simulink model "sml_trajectory"  (R2016a)
settings: Solver=VariableStepAuto  StartTime=0.0  StopTime=10.0  RelTol=1e-3
libraries: simulink x2
settings Model: Creator=Duy Nam  LastModifiedBy=Duy Nam

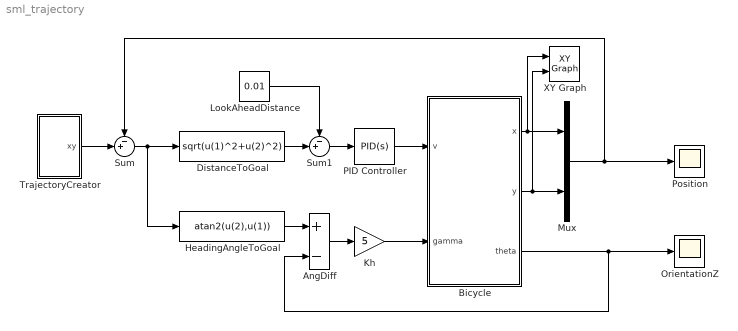
== system sml_trajectory ==
  AngDiff : Sum  Inputs=+-
  Bicycle : Subsystem
  DistanceToGoal : Fcn  Expr=sqrt(u(1)^2+u(2)^2)
  HeadingAngleToGoal : Fcn  Expr=atan2(u(2),u(1))
  Kh : Gain  Gain=5
  LookAheadDistance : Constant  Value=0.01
  Mux : Mux  Inputs=2
  OrientationZ : Scope
  PID Controller : simulink/Continuous/PID Controller  Controller=PID  TimeDomain=Continuous-time  SampleTime=-1  IntegratorMethod=Forward Euler  FilterMethod=Forward Euler  Form=Parallel  UseFilter=on  ControllerParametersSource=internal  P=4  I=0.5  D=0  N=100  InitialConditionSource=internal  InitialConditionForIntegrator=0  InitialConditionForFilter=0  ExternalReset=none  LimitOutput=off  UpperSaturationLimit=inf  LowerSaturationLimit=-inf  LinearizeAsGain=on  AntiWindupMode=none  Kb=1  TrackingMode=off  Kt=1  PParamMin=[]  PParamMax=[]  IParamMin=[]  IParamMax=[]  DParamMin=[]  DParamMax=[]  NParamMin=[]  NParamMax=[]  KbParamMin=[]  KbParamMax=[]  KtParamMin=[]  KtParamMax=[]  POutMin=[]  POutMax=[]  IOutMin=[]  IOutMax=[]  DOutMin=[]  DOutMax=[]  NOutMin=[]  NOutMax=[]  KbOutMin=[]  KbOutMax=[]  KtOutMin=[]  KtOutMax=[]  IntegratorOutMin=[]  IntegratorOutMax=[]  FilterOutMin=[]  FilterOutMax=[]  SumOutMin=[]  SumOutMax=[]  SumI1OutMin=[]  SumI1OutMax=[]  SumI2OutMin=[]  SumI2OutMax=[]  SumI3OutMin=[]  SumI3OutMax=[]  SumDOutMin=[]  SumDOutMax=[]  SaturationOutMin=[]  SaturationOutMax=[]  IntegratorContinuousStateAttributes=''  IntegratorStateMustResolveToSignalObject=off  IntegratorRTWStateStorageClass=Auto  FilterContinuousStateAttributes=''  FilterStateMustResolveToSignalObject=off  FilterRTWStateStorageClass=Auto  DifferentiatorICPrevScaledInput=0  DifferentiatorOutMin=[]  DifferentiatorOutMax=[]
  Position : Scope
  Sum : Sum  Inputs=-+|
  Sum1 : Sum  Inputs=-+|
  TrajectoryCreator : Subsystem
  XY Graph : simulink/Sinks/XY Graph  xmin=-5  xmax=5  ymin=-5  ymax=5  st=-1
  wires:
  Bicycle/1(x) -> XY Graph/1, Mux/1
  Bicycle/2(y) -> XY Graph/2, Mux/2
  Bicycle/3(theta) -> AngDiff/2, OrientationZ/1
  Mux/1 -> Sum/1, Position/1
  Sum/1 -> HeadingAngleToGoal/1, DistanceToGoal/1
  DistanceToGoal/1 -> Sum1/2
  LookAheadDistance/1 -> Sum1/1
  HeadingAngleToGoal/1 -> AngDiff/1
  Sum1/1 -> PID Controller/1
  AngDiff/1 -> Kh/1
  Kh/1 -> Bicycle/2(gamma)
  PID Controller/1 -> Bicycle/1(v)
  TrajectoryCreator/1(xy) -> Sum/2

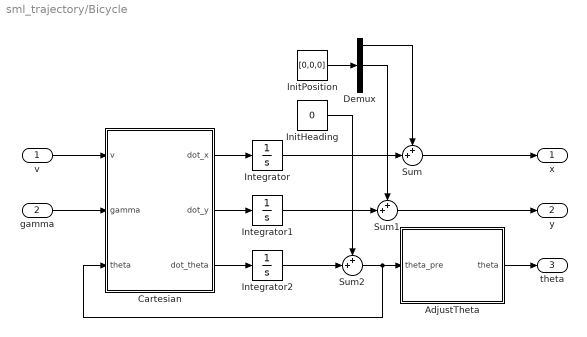
== system sml_trajectory/Bicycle ==
  v : Inport
  gamma : Inport  Port=2
  AdjustTheta : MATLAB Function  TreatAsAtomicUnit=on
  Cartesian : MATLAB Function  TreatAsAtomicUnit=on
  Demux : Demux  Outputs=3
  InitHeading : Constant  Value=0
  InitPosition : Constant  Value=[0,0,0]
  Integrator : Integrator
  Integrator1 : Integrator
  Integrator2 : Integrator
  Sum : Sum  Inputs=++|
  Sum1 : Sum  Inputs=++|
  Sum2 : Sum  Inputs=++|
  x : Outport
  y : Outport  Port=2
  theta : Outport  Port=3
  wires:
  Cartesian/1(dot_x) -> Integrator/1
  Integrator/1 -> Sum/2
  Cartesian/2(dot_y) -> Integrator1/1
  Integrator1/1 -> Sum1/2
  Cartesian/3(dot_theta) -> Integrator2/1
  AdjustTheta/1(theta) -> theta/1
  Sum2/1 -> Cartesian/3(theta), AdjustTheta/1(theta_pre)
  v/1 -> Cartesian/1(v)
  gamma/1 -> Cartesian/2(gamma)
  InitPosition/1 -> Demux/1
  Sum/1 -> x/1
  Demux/1 -> Sum/1
  Sum1/1 -> y/1
  Demux/2 -> Sum1/1
  Integrator2/1 -> Sum2/2
  InitHeading/1 -> Sum2/1

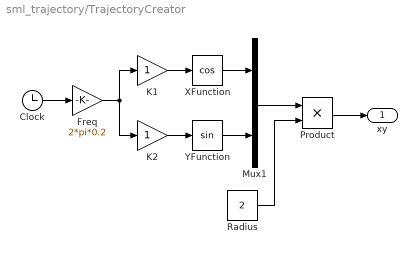
== system sml_trajectory/TrajectoryCreator ==
  Clock : Clock
  Freq : Gain  Gain=2*pi*0.2
  K1 : Gain
  K2 : Gain
  Mux1 : Mux  Inputs=2
  Product : Product
  Radius : Constant  Value=2
  XFunction : Trigonometry  Operator=cos
  YFunction : Trigonometry
  xy : Outport
  wires:
  XFunction/1 -> Mux1/1
  YFunction/1 -> Mux1/2
  K2/1 -> YFunction/1
  Mux1/1 -> Product/1
  Freq/1 -> K1/1, K2/1
  Clock/1 -> Freq/1
  Radius/1 -> Product/2
  Product/1 -> xy/1
  K1/1 -> XFunction/1

== matlab function sml_trajectory/Bicycle/AdjustTheta ==
  data: theta_pre input; theta output
function theta = AdjustTheta(theta_pre)
% ADJUSTTHETA Adjust the heading angle always between [-pi/2;pi/2]
%% INPUTS
% theta_pre = The heading angle before adjust
%% OUTPUTS
% theta = The heading angle after adjust
%% Adjust Theta
theta = theta_pre - 2*pi*floor((theta_pre + pi)/(2*pi));
end

== matlab function sml_trajectory/Bicycle/Cartesian ==
  data: dot_x output; dot_y output; v input; gamma input; theta input; dot_theta output
function [dot_x, dot_y, dot_theta] = Cartesian(v, gamma, theta)
% CARTESIAN Compute the velocity of robot in world frame
%% INPUTS
% v     = The velocity of the back wheel
% gamma = The steering wheel angle
% theta = The heading angle
%% OUTPUTS
% dot_x     = The velocity of robot in world frame x-axis
% dot_y     = The velocity of robot in world frame y-axis
% dot_theta = The rate of change of heading
%% Parameters
L = params_bicycle();
%% Cartesian
dot_x = v*cos(theta);
dot_y = v*sin(theta);
dot_theta = v/L*tan(gamma);
end
